simulink subsystem "FeedforwardcompensatorPID"  (R2024b)
settings: Solver=VariableStepAuto  StartTime=0.0  StopTime=10.0  RelTol=1e-3
values from neighbouring files (symbols this model uses):
  Beq = 1.0459e-06    [Plant_EstimTrialUpdateLAB17_04_25.m]
  Jeq = 9.8651e-07    [Plant_EstimTrialUpdateLAB17_04_25.m]
  kdrv = 0.6    [Plant_EstimTrialUpdateLAB17_04_25.m]
  ke = 7.68 * 0.001    (= 0.00768)    [Plant_EstimTrialUpdateLAB17_04_25.m]
  Kt = 1.088 * ozin2Nm    (= 0.00768128)    [Plant_EstimTrialUpdateLAB17_04_25.m]
  N = 14    [Plant_EstimTrialUpdateLAB17_04_25.m]
  Req = Ra + Rs    (= 3.1)    [Plant_EstimTrialUpdateLAB17_04_25.m]
  tausf = 0.0061    [Plant_EstimTrialUpdateLAB17_04_25.m]
settings Model: Creator=Utente  LastModifiedBy=Buton

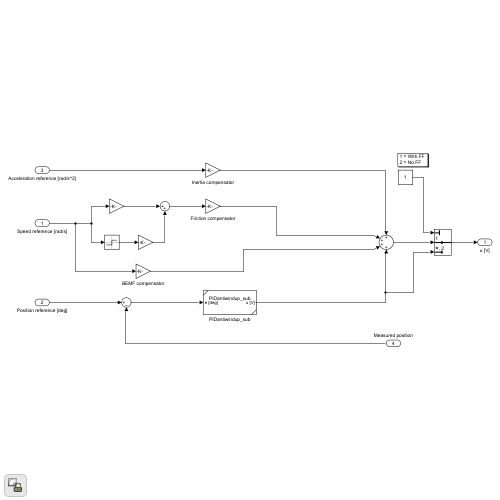
[thumbnail: Simulink's stored preview of the top-level diagram]
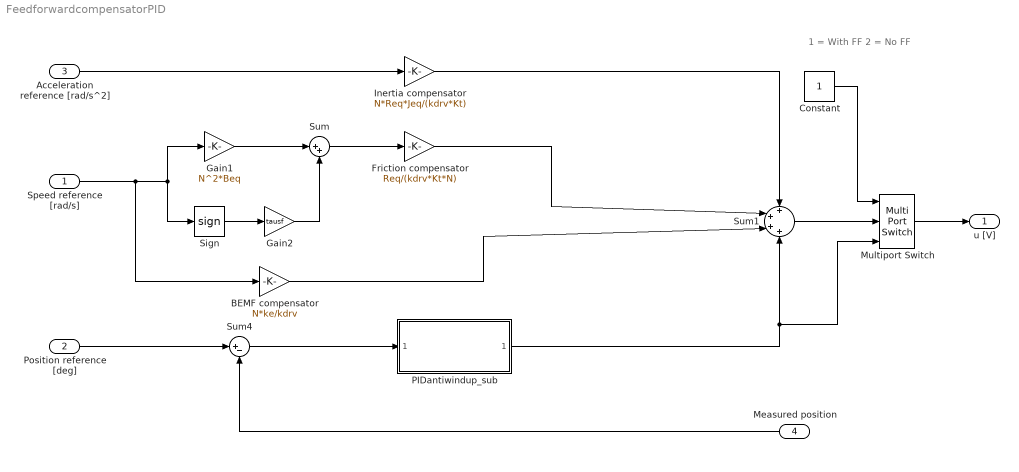
== system FeedforwardcompensatorPID ==
  note: 1 = With FF
      | 2 = No FF
  Speed reference [rad/s] : Inport
  Position reference [deg] : Inport  Port=2
  Acceleration reference [rad/s^2] : Inport  Port=3
  Measured position : Inport  Port=4
  BEMF compensator : Gain  Gain=N*ke/kdrv
  Constant : Constant
  Friction compensator : Gain  Gain=Req/(kdrv*Kt*N)
  Gain1 : Gain  Gain=N^2*Beq
  Gain2 : Gain  Gain=tausf
  Inertia compensator : Gain  Gain=N*Req*Jeq/(kdrv*Kt)
  Multiport Switch : MultiPortSwitch  Inputs=2  SaturateOnIntegerOverflow=off  InputSameDT=off
  PIDantiwindup_sub : Subsystem  ReferencedSubsystem=PIDantiwindup_sub
  Sign : Signum
  Sum : Sum  Inputs=|++
  Sum1 : Sum  Inputs=++++
  Sum4 : Sum  Inputs=|+-
  u [V] : Outport
  wires:
  Sign/1 -> Gain2/1
  Gain2/1 -> Sum/2
  Gain1/1 -> Sum/1
  Sum/1 -> Friction compensator/1
  Speed reference [rad/s]/1 -> BEMF compensator/1, Sign/1, Gain1/1
  Position reference [deg]/1 -> Sum4/1
  Measured position/1 -> Sum4/2
  Sum4/1 -> PIDantiwindup_sub/1
  BEMF compensator/1 -> Sum1/3
  Friction compensator/1 -> Sum1/2
  Inertia compensator/1 -> Sum1/1
  Sum1/1 -> Multiport Switch/2
  PIDantiwindup_sub/1 -> Multiport Switch/3, Sum1/4
  Constant/1 -> Multiport Switch/1
  Multiport Switch/1 -> u [V]/1
  Acceleration reference [rad/s^2]/1 -> Inertia compensator/1
